simulink library "commeqprivlib"  (Simulink 6.0)
settings: Solver=ode45  SolverMode=SingleTasking  StartTime=0.0  StopTime=10.0  RelTol=1e-3
undefined symbols (not defined in the file or in its folder): bias, delay, incMu, lambda, leakage, maxMu, minMu, nFwdTaps, nSamp, nTaps, Rows, sigConst, stepSize
libraries: commeqprivlib x11, dspsigattribs x9, dspsigops x8, simulink x7, dspmtrx3 x5, dspindex x2, dspsrcs4 x2, dspbuff3 x1, dspstat3 x1
settings Model: Creator=skeene  LastModifiedBy=mclark  ProdHWDeviceType=Specified
settings DataIOCC: SignalLoggingName=logsOut
settings OptimizationCC: BooleanDataType=off
settings DebuggingCC: CheckExecutionContextPreStartOutputMsg=on  CheckExecutionContextRuntimeOutputMsg=on  SolverPrmCheckMsg=none
settings HardwareCC: ProdHWDeviceType=Specified  TargetUnknown=on
settings ModelReferenceCC: UpdateModelReferenceTargets=IfOutOfDate
settings GRTTargetCC: LifeSpan=inf
settings SFSimCC: SFSimApplyToAllLibs=on  SFSimBuildMode=Incremental

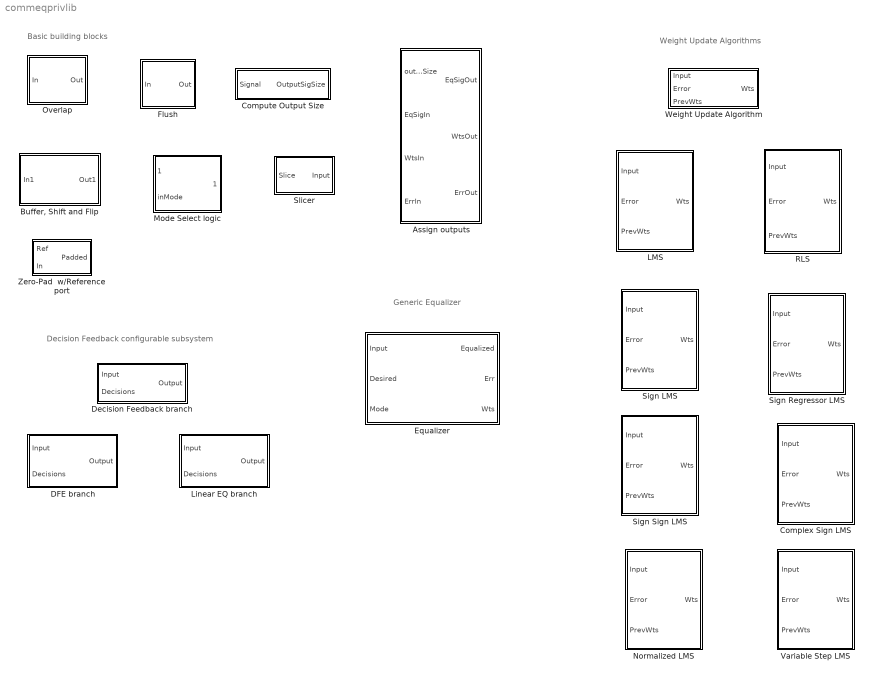
== system commeqprivlib ==
  note: Basic building blocks
  note: Decision Feedback configurable subsystem
  note: Generic Equalizer
  note: Weight Update Algorithms
  Assign outputs : Subsystem  EnableExecutionContextPropagation=on
  "Buffer, Shift and Flip" : Subsystem  EnableExecutionContextPropagation=on
  Complex Sign LMS : Subsystem  EnableExecutionContextPropagation=on
  Compute Output Size : Subsystem  EnableExecutionContextPropagation=on
  DFE branch : Subsystem  EnableExecutionContextPropagation=on
  Decision Feedback branch : Subsystem  BlockChoice=DFE branch  EnableExecutionContextPropagation=on
      settings: TemplateBlock=self  MemberBlocks=DFE branch,Linear EQ branch
  "Equalizer " : Subsystem  EnableExecutionContextPropagation=on  mask{eqType=Linear, alg=LMS}
      mask prompts: eqType "Equalizer type"; alg "Weight update algorithm"
      mask init:
      | commblkeq
      mask StyleString: popup(Linear|DFE),popup(LMS|RLS|Sign LMS|Sign Regressor LMS|Sign Sign LMS|Complex Sign LMS|Normalized LMS|Variable Step LMS)
      mask CallbackString: commblkeq|commblkeq
  Flush : Subsystem  EnableExecutionContextPropagation=on
  LMS : Subsystem  EnableExecutionContextPropagation=on
  Linear EQ branch : Subsystem  EnableExecutionContextPropagation=on
  Mode Select logic : Subsystem  EnableExecutionContextPropagation=on
  Normalized LMS : Subsystem  EnableExecutionContextPropagation=on
  Overlap : Subsystem  EnableExecutionContextPropagation=on
  RLS : Subsystem  EnableExecutionContextPropagation=on
  Sign LMS : Subsystem  EnableExecutionContextPropagation=on
  Sign Regressor LMS : Subsystem  EnableExecutionContextPropagation=on
  Sign Sign LMS : Subsystem  EnableExecutionContextPropagation=on
  Slicer : Subsystem  Orientation=left  EnableExecutionContextPropagation=on
  Variable Step LMS : Subsystem  EnableExecutionContextPropagation=on
  Weight Update Algorithm : Subsystem  BlockChoice=LMS  EnableExecutionContextPropagation=on
      settings: TemplateBlock=self  MemberBlocks=Complex Sign LMS,LMS,Normalized LMS,RLS,Sign LMS,Sign Regressor LMS,Sign Sign LMS,Variable Step LMS
  Zero-Pad  w/Reference port : Subsystem  EnableExecutionContextPropagation=on

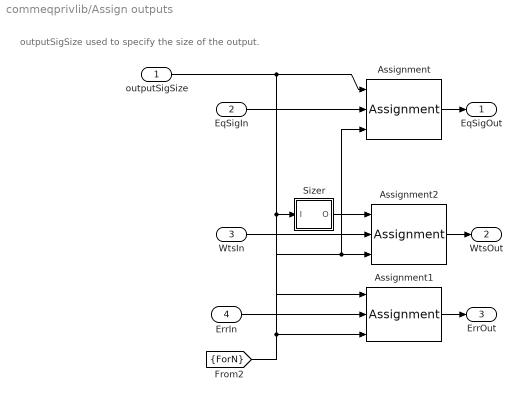
== system commeqprivlib/Assign outputs ==
  note: outputSigSize used to specify
      | the size of the output.
  outputSigSize : Inport  LatchInput=off
  EqSigIn : Inport  Port=2  LatchInput=off
  WtsIn : Inport  Port=3  LatchInput=off
  ErrIn : Inport  Port=4  LatchInput=off
  Assignment : Assignment  IndexMode=Zero-based  ElementSrc=External  Rows=-1  ColumnSrc=External  DiagnosticForDimensions=Error
  Assignment1 : Assignment  IndexMode=Zero-based  ElementSrc=External  Rows=-1  ColumnSrc=External  DiagnosticForDimensions=Error
  Assignment2 : Assignment  InputType=Matrix  IndexMode=Zero-based  ElementSrc=External  Rows=-1  ColumnSrc=External  DiagnosticForDimensions=Error
  Sizer : Subsystem  EnableExecutionContextPropagation=on
  EqSigOut : Outport
  WtsOut : Outport  Port=2
  ErrOut : Outport  Port=3
  wires:
  outputSigSize/1 -> Sizer/1(I), Assignment1/1, Assignment/1
  [ForN] -> Assignment1/3, Assignment/3, Assignment2/3
  Sizer/1(O) -> Assignment2/1
  EqSigIn/1 -> Assignment/2
  WtsIn/1 -> Assignment2/2
  ErrIn/1 -> Assignment1/2
  Assignment/1 -> EqSigOut/1
  Assignment2/1 -> WtsOut/1
  Assignment1/1 -> ErrOut/1

== system commeqprivlib/Buffer, Shift and Flip ==
  In1 : Inport  LatchInput=off
  Bias1 : Bias  Bias=0:nFwdTaps-1
  Flip : dspindex/Flip  dim=Columns
  Frame Status Conversion : dspsigattribs/Frame Status Conversion  growRefPort=off  outframe=Sample-based
  Gain : Gain  Gain=nSamp  SaturateOnIntegerOverflow=on
  Selector : Selector  IndexMode=Zero-based  ElementSrc=External  Elements=[1 3]
  Out1 : Outport
  wires:
  Frame Status Conversion/1 -> Out1/1
  In1/1 -> Selector/1
  Gain/1 -> Bias1/1
  [ForN] -> Gain/1
  Selector/1 -> Flip/1
  Flip/1 -> Frame Status Conversion/1
  Bias1/1 -> Selector/2

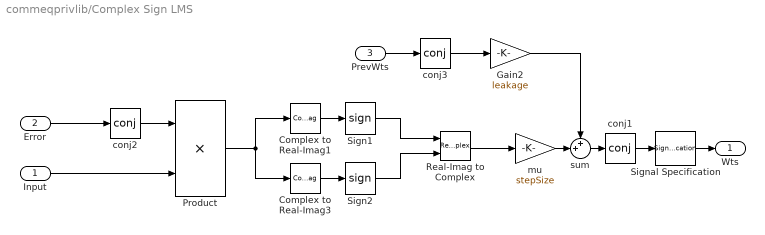
== system commeqprivlib/Complex Sign LMS ==
  Input : Inport  LatchInput=off
  Error : Inport  Port=2  LatchInput=off
  PrevWts : Inport  Port=3  LatchInput=off
  Complex to Real-Imag1 : ComplexToRealImag  Output=Real
  Complex to Real-Imag3 : ComplexToRealImag  Output=Imag
  Gain2 : Gain  Gain=leakage  SaturateOnIntegerOverflow=on
  Product : Product  SaturateOnIntegerOverflow=on
  Real-Imag to Complex : RealImagToComplex
  Sign1 : Signum
  Sign2 : Signum
  Signal Specification : SignalSpecification
      settings: SignalType=complex
  conj1 : Math  Operator=conj  SaturateOnIntegerOverflow=on
  conj2 : Math  Operator=conj  SaturateOnIntegerOverflow=on
  conj3 : Math  Operator=conj  SaturateOnIntegerOverflow=on
  mu : Gain  Gain=stepSize  SaturateOnIntegerOverflow=on
  sum : Sum  Inputs=++|  SaturateOnIntegerOverflow=on  InputSameDT=on
  Wts : Outport  InitialOutput=0
  wires:
  Product/1 -> Complex to Real-Imag1/1, Complex to Real-Imag3/1
  Complex to Real-Imag1/1 -> Sign1/1
  Gain2/1 -> sum/1
  PrevWts/1 -> conj3/1
  sum/1 -> conj1/1
  Input/1 -> Product/2
  Error/1 -> conj2/1
  mu/1 -> sum/2
  conj1/1 -> Signal Specification/1
  conj3/1 -> Gain2/1
  conj2/1 -> Product/1
  Signal Specification/1 -> Wts/1
  Real-Imag to Complex/1 -> mu/1
  Sign1/1 -> Real-Imag to Complex/1
  Complex to Real-Imag3/1 -> Sign2/1
  Sign2/1 -> Real-Imag to Complex/2

== system commeqprivlib/Compute Output Size ==
  Signal : Inport  LatchInput=off
  Downsample : dspsigops/Downsample  N=nSamp  phase=0  ic=0  smode=Force single rate  fmode=Maintain input frame rate
  Submatrix : dspmtrx3/Submatrix  RowSpan=Range of rows  RowStartMode=First  RowStartIndex=1  RowEndMode=Offset from last  RowEndIndex=nFwdTaps  ColSpan=Range of columns  ColStartMode=First  ColStartIndex=1  ColEndMode=Last  ColEndIndex=1
  OutputSigSize : Outport
  wires:
  Downsample/1 -> OutputSigSize/1
  Submatrix/1 -> Downsample/1
  Signal/1 -> Submatrix/1

== system commeqprivlib/DFE branch ==
  Input : Inport  LatchInput=off
  Decisions : Inport  Orientation=up  Port=2  LatchInput=off
  Delay Line : dspbuff3/Delay Line  Orientation=up  siz=nFdbkTaps  ic=0  directfeed=off
  Flip1 : dspindex/Flip  Orientation=up  dim=Columns
  Matrix Concatenation : simulink/Math Operations/Matrix Concatenation  numInports=2  catMethod=Vertical
  Output : Outport
  wires:
  Matrix Concatenation/1 -> Output/1
  Input/1 -> Matrix Concatenation/1
  Decisions/1 -> Delay Line/1
  Delay Line/1 -> Flip1/1
  Flip1/1 -> Matrix Concatenation/2

== system commeqprivlib/Decision Feedback branch ==
  Input : Inport  LatchInput=off
  Decisions : Inport  Port=2  LatchInput=off
  DFE branch : commeqprivlib/DFE branch  SimViewingDevice=off  DataTypeOverride=UseLocalSettings  MinMaxOverflowLogging=UseLocalSettings
      settings: Permissions=ReadWrite  RTWFcnNameOpts=Auto  RTWFileNameOpts=Auto
  Output : Outport
  wires:
  Input/1 -> DFE branch/1
  Decisions/1 -> DFE branch/2
  DFE branch/1 -> Output/1

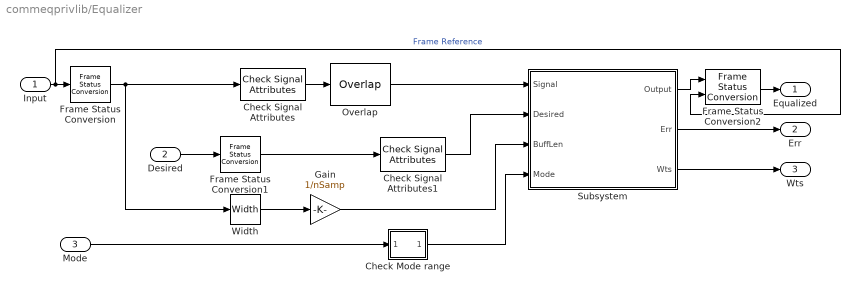
== system commeqprivlib/Equalizer  ==
  Input : Inport  LatchInput=off
  Desired : Inport  Port=2  LatchInput=off
  Mode : Inport  Port=3  LatchInput=off
  Check Mode range : Subsystem  EnableExecutionContextPropagation=on
  Check Signal Attributes : dspsigattribs/Check Signal Attributes  SigAttribCheckMethod=Does not match attributes exactly  Complexity=Complex  Frame=Ignore  DimsCheckMethod=Is not...  Dimensions=Full matrix (2-D)  DatatypeCheckMethod=Ignore  DatatypeGeneral=Boolean  DtypeFloatSpecific=Any floating-point  DtypeFixedSpecific=Any fixed-point  DtypeIntSpecific=Any integer  SampleMode=Ignore
  Check Signal Attributes1 : dspsigattribs/Check Signal Attributes  SigAttribCheckMethod=Does not match attributes exactly  Complexity=Complex  Frame=Ignore  DimsCheckMethod=Is not...  Dimensions=Full matrix (2-D)  DatatypeCheckMethod=Ignore  DatatypeGeneral=Boolean  DtypeFloatSpecific=Any floating-point  DtypeFixedSpecific=Any fixed-point  DtypeIntSpecific=Any integer  SampleMode=Ignore
  Frame Status Conversion : dspsigattribs/Frame Status Conversion  growRefPort=off  outframe=Frame-based
  Frame Status Conversion1 : dspsigattribs/Frame Status Conversion  growRefPort=off  outframe=Frame-based
  Frame Status Conversion2 : dspsigattribs/Frame Status Conversion  growRefPort=on  outframe=Frame-based
  Gain : Gain  Gain=1/nSamp  SaturateOnIntegerOverflow=on
  Overlap : commeqprivlib/Overlap
  Subsystem : Subsystem  EnableExecutionContextPropagation=on
  Width : Width  ShowAdditionalParam=on
  Equalized : Outport
  Err : Outport  Port=2
  Wts : Outport  Port=3
  wires:
  Frame Status Conversion/1 -> Width/1, Check Signal Attributes/1
  Frame Status Conversion1/1 -> Check Signal Attributes1/1
  Frame Status Conversion2/1 -> Equalized/1
  Subsystem/1(Output) -> Frame Status Conversion2/1
  Check Mode range/1("  ") -> Subsystem/4(Mode)
  Subsystem/3(Wts) -> Wts/1
  Subsystem/2(Err) -> Err/1
  Mode/1 -> Check Mode range/1("        ")
  Gain/1 -> Subsystem/3(BuffLen)
  Overlap/1 -> Subsystem/1(Signal)
  Desired/1 -> Frame Status Conversion1/1
  Input/1 -> Frame Status Conversion/1, Frame Status Conversion2/2  "Frame Reference"
  Width/1 -> Gain/1
  Check Signal Attributes1/1 -> Subsystem/2(Desired)
  Check Signal Attributes/1 -> Overlap/1

== system commeqprivlib/Flush ==
  note: This subsytem appends delay
      | samples to the reference signal.
      | The purpose of this is to flush out the
      | final samples from the delay block
      | that follows this subsystem.
  In : Inport  LatchInput=off
  Delay2 : dspsigops/Delay  Orientation=left  dly_unit=Samples  delay=delay  ic_detail=off  dif_ic_for_ch=off  dif_ic_for_dly=off  ic=0  reset_popup=None
  Matrix Concatenation : simulink/Math Operations/Matrix Concatenation  numInports=2  catMethod=Vertical
  Signal Specification : simulink/Signal Attributes/Signal Specification  Orientation=up  D=[delay 1]  Ts=-1  DataType=auto  OutDataType=sfix(16)  OutScaling=2^0
      settings: SignalType=auto  SamplingMode=auto
  Submatrix : dspmtrx3/Submatrix  Orientation=down  RowSpan=Range of rows  RowStartMode=Offset from last  RowStartIndex=delay-1  RowEndMode=Last  RowEndIndex=1  ColSpan=Range of columns  ColStartMode=First  ColStartIndex=1  ColEndMode=Last  ColEndIndex=1
  Out : Outport
  wires:
  Submatrix/1 -> Delay2/1
  Delay2/1 -> Signal Specification/1
  Matrix Concatenation/1 -> Out/1, Submatrix/1
  In/1 -> Matrix Concatenation/1
  Signal Specification/1 -> Matrix Concatenation/2

== system commeqprivlib/LMS ==
  Input : Inport  LatchInput=off
  Error : Inport  Port=2  LatchInput=off
  PrevWts : Inport  Port=3  LatchInput=off
  Gain2 : Gain  Gain=leakage  SaturateOnIntegerOverflow=on
  Product : Product  SaturateOnIntegerOverflow=on
  conj : Math  Operator=conj  SaturateOnIntegerOverflow=on
  mu : Gain  Gain=stepSize  SaturateOnIntegerOverflow=on
  sum : Sum  Inputs=++|  SaturateOnIntegerOverflow=on  InputSameDT=on
  Wts : Outport  InitialOutput=0
  wires:
  mu/1 -> Product/1
  Error/1 -> mu/1
  conj/1 -> Product/2
  Input/1 -> conj/1
  sum/1 -> Wts/1
  Product/1 -> sum/2
  PrevWts/1 -> Gain2/1
  Gain2/1 -> sum/1

== system commeqprivlib/Linear EQ branch ==
  note: There is no feedback in a linear equalizer
  Input : Inport  LatchInput=off
  Decisions : Inport  Orientation=up  Port=2  LatchInput=off
  Terminator : Terminator
      settings: Orientation=up
  Output : Outport
  wires:
  Decisions/1 -> Terminator/1
  Input/1 -> Output/1

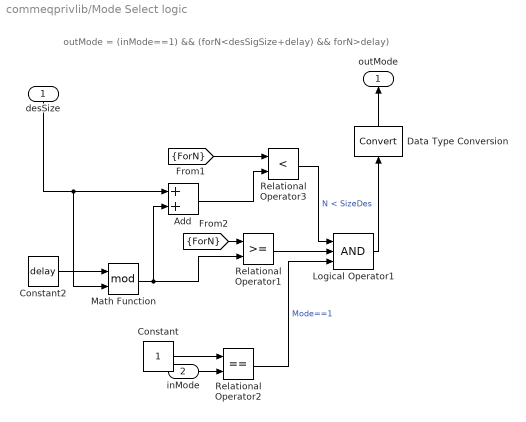
== system commeqprivlib/Mode Select logic ==
  note: outMode = (inMode==1) && (forN<desSigSize+delay) && forN>delay)
  desSize : Inport  Orientation=down  LatchInput=off
  inMode : Inport  Port=2  LatchInput=off
  Add : Sum  OutScaling=2^-10
  Constant : Constant
  Constant2 : Constant  Value=delay
  Data Type Conversion : DataTypeConversion  Orientation=up  OutDataTypeMode=double
  Logical Operator1 : Logic  Inputs=3  AllPortsSameDT=off  OutDataTypeMode=Boolean
  Math Function : Math  Operator=mod  SaturateOnIntegerOverflow=on
  Relational Operator1 : RelationalOperator  LogicOutDataTypeMode=Boolean
  Relational Operator2 : RelationalOperator  Operator===  LogicOutDataTypeMode=Boolean
  Relational Operator3 : RelationalOperator  Operator=<  LogicOutDataTypeMode=Boolean
  outMode : Outport  Orientation=up
  wires:
  inMode/1 -> Relational Operator2/2
  desSize/1 -> Add/1, Math Function/2
  Data Type Conversion/1 -> outMode/1
  Logical Operator1/1 -> Data Type Conversion/1
  Relational Operator3/1 -> Logical Operator1/1  "N < SizeDes"
  [ForN] -> Relational Operator3/1
  Constant/1 -> Relational Operator2/1
  Relational Operator2/1 -> Logical Operator1/3  "Mode==1"
  [ForN] -> Relational Operator1/1
  Relational Operator1/1 -> Logical Operator1/2
  Add/1 -> Relational Operator3/2
  Math Function/1 -> Add/2, Relational Operator1/2
  Constant2/1 -> Math Function/1

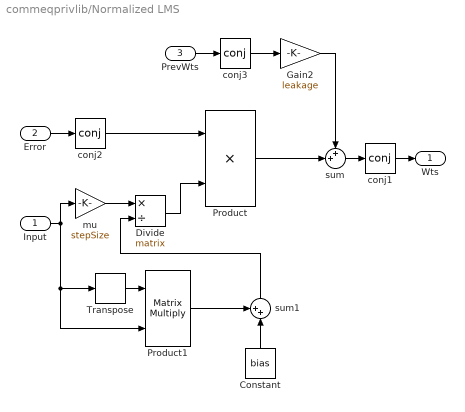
== system commeqprivlib/Normalized LMS ==
  Input : Inport  LatchInput=off
  Error : Inport  Port=2  LatchInput=off
  PrevWts : Inport  Port=3  LatchInput=off
  Constant : Constant  Orientation=up  Value=bias
  Divide : Product  Inputs=*/  Multiplication=Matrix(*)  OutScaling=2^-10
  Gain2 : Gain  Gain=leakage  SaturateOnIntegerOverflow=on
  Product : Product  SaturateOnIntegerOverflow=on
  Product1 : Product  Multiplication=Matrix(*)  SaturateOnIntegerOverflow=on
  Transpose : dspmtrx3/Transpose  Hermitian=on
  conj1 : Math  Operator=conj  SaturateOnIntegerOverflow=on
  conj2 : Math  Operator=conj  SaturateOnIntegerOverflow=on
  conj3 : Math  Operator=conj  SaturateOnIntegerOverflow=on
  mu : Gain  Gain=stepSize  SaturateOnIntegerOverflow=on
  sum : Sum  Inputs=++|  SaturateOnIntegerOverflow=on  InputSameDT=on
  sum1 : Sum  Orientation=up  Inputs=++|  SaturateOnIntegerOverflow=on  InputSameDT=on
  Wts : Outport  InitialOutput=0
  wires:
  conj1/1 -> Wts/1
  conj3/1 -> Gain2/1
  Error/1 -> conj2/1
  sum/1 -> conj1/1
  Product/1 -> sum/2
  PrevWts/1 -> conj3/1
  Gain2/1 -> sum/1
  conj2/1 -> Product/1
  Transpose/1 -> Product1/1
  Input/1 -> Product1/2, Transpose/1, mu/1
  Constant/1 -> sum1/2
  Product1/1 -> sum1/1
  sum1/1 -> Divide/2
  Divide/1 -> Product/2
  mu/1 -> Divide/1

== system commeqprivlib/Overlap ==
  note: This subsystem appends nTaps samples
      | to the input signal. The purpose of this is to remember
      | the previous nTaps sampes, as they are needed to
      | compute the current weights.
  In : Inport  LatchInput=off
  Delay2 : dspsigops/Delay  Orientation=left  dly_unit=Samples  delay=nFwdTaps  ic_detail=off  dif_ic_for_ch=off  dif_ic_for_dly=off  ic=0  reset_popup=None
  Matrix Concatenation : simulink/Math Operations/Matrix Concatenation  numInports=2  catMethod=Vertical
  Signal Specification : simulink/Signal Attributes/Signal Specification  Orientation=down  D=[nFwdTaps 1]  Ts=-1  DataType=auto  OutDataType=sfix(16)  OutScaling=2^0
      settings: SignalType=auto  SamplingMode=auto
  Submatrix : dspmtrx3/Submatrix  Orientation=up  RowSpan=Range of rows  RowStartMode=Offset from last  RowStartIndex=nFwdTaps-1  RowEndMode=Last  RowEndIndex=1  ColSpan=Range of columns  ColStartMode=First  ColStartIndex=1  ColEndMode=Last  ColEndIndex=1
  Out : Outport
  wires:
  In/1 -> Matrix Concatenation/2
  Submatrix/1 -> Delay2/1
  Delay2/1 -> Signal Specification/1
  Matrix Concatenation/1 -> Out/1, Submatrix/1
  Signal Specification/1 -> Matrix Concatenation/1

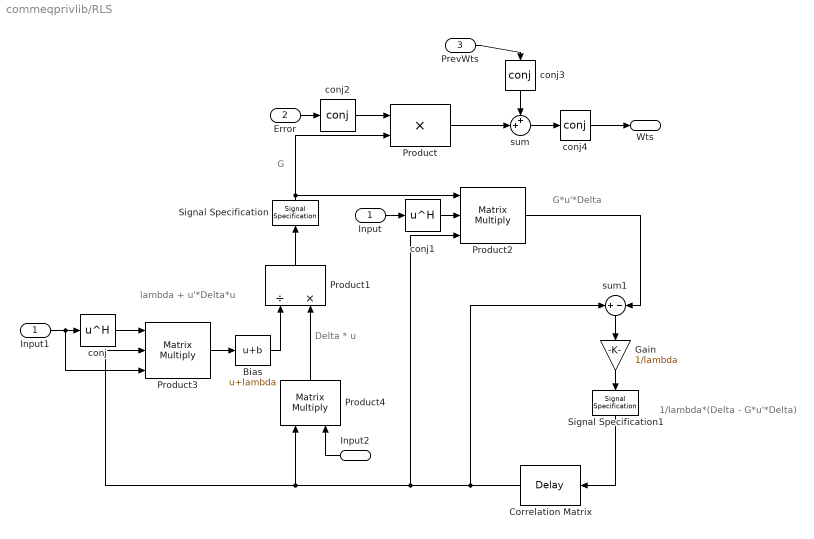
== system commeqprivlib/RLS ==
  note: G
  note: lambda + u'*Delta*u
  note: G*u'*Delta
  note: 1/lambda*(Delta - G*u'*Delta)
  note: Delta * u
  Input : Inport  LatchInput=off
  Error : Inport  Port=2  LatchInput=off
  PrevWts : Inport  Port=3  LatchInput=off
  Bias : Bias  Bias=lambda
  Correlation Matrix : dspsigops/Delay  Orientation=left  dly_unit=Samples  delay=1  ic_detail=on  dif_ic_for_ch=on  dif_ic_for_dly=off  ic=invCorr  reset_popup=None
  Gain : Gain  Orientation=down  Gain=1/lambda
  Input1 : InportShadow  LatchInput=off
  Input2 : InportShadow  Orientation=left  LatchInput=off
  Product : Product  SaturateOnIntegerOverflow=on
  Product1 : Product  Orientation=up  Inputs=/*  SaturateOnIntegerOverflow=on
  Product2 : Product  Inputs=3  Multiplication=Matrix(*)  SaturateOnIntegerOverflow=on
  Product3 : Product  Inputs=3  Multiplication=Matrix(*)  SaturateOnIntegerOverflow=on
  Product4 : Product  Orientation=up  Multiplication=Matrix(*)  SaturateOnIntegerOverflow=on
  Signal Specification : SignalSpecification  Orientation=up  Dimensions=[nTaps 1]
  Signal Specification1 : SignalSpecification  Orientation=down  Dimensions=[nTaps nTaps]
  conj : Math  Operator=hermitian  SaturateOnIntegerOverflow=on
  conj1 : Math  Operator=hermitian  SaturateOnIntegerOverflow=on
  conj2 : Math  Operator=conj  SaturateOnIntegerOverflow=on
  conj3 : Math  Orientation=down  Operator=conj  SaturateOnIntegerOverflow=on
  conj4 : Math  Operator=conj  SaturateOnIntegerOverflow=on
  sum : Sum  Inputs=++|  SaturateOnIntegerOverflow=on  InputSameDT=on
  sum1 : Sum  Orientation=down  Inputs=+-  SaturateOnIntegerOverflow=on  InputSameDT=on
  Wts : Outport  InitialOutput=0
  wires:
  Error/1 -> conj2/1
  Product1/1 -> Signal Specification/1
  Product/1 -> sum/2
  PrevWts/1 -> conj3/1
  sum/1 -> conj4/1
  Input/1 -> conj1/1
  conj/1 -> Product3/1
  Input1/1 -> conj/1, Product3/3
  Product3/1 -> Bias/1
  Bias/1 -> Product1/1
  Product4/1 -> Product1/2
  Input2/1 -> Product4/2
  Correlation Matrix/1 -> Product4/1, Product3/2, Product2/3, sum1/1
  Product2/1 -> sum1/2
  sum1/1 -> Gain/1
  Gain/1 -> Signal Specification1/1
  conj1/1 -> Product2/2
  conj2/1 -> Product/1
  Signal Specification/1 -> Product/2, Product2/1
  Signal Specification1/1 -> Correlation Matrix/1
  conj3/1 -> sum/1
  conj4/1 -> Wts/1

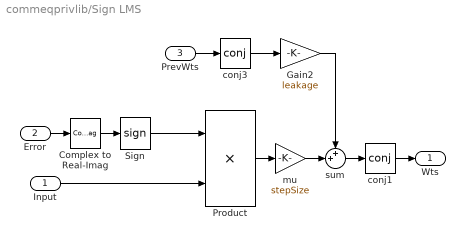
== system commeqprivlib/Sign LMS ==
  Input : Inport  LatchInput=off
  Error : Inport  Port=2  LatchInput=off
  PrevWts : Inport  Port=3  LatchInput=off
  Complex to Real-Imag : ComplexToRealImag  Output=Real
  Gain2 : Gain  Gain=leakage  SaturateOnIntegerOverflow=on
  Product : Product  SaturateOnIntegerOverflow=on
  Sign : Signum
  conj1 : Math  Operator=conj  SaturateOnIntegerOverflow=on
  conj3 : Math  Operator=conj  SaturateOnIntegerOverflow=on
  mu : Gain  Gain=stepSize  SaturateOnIntegerOverflow=on
  sum : Sum  Inputs=++|  SaturateOnIntegerOverflow=on  InputSameDT=on
  Wts : Outport  InitialOutput=0
  wires:
  Gain2/1 -> sum/1
  PrevWts/1 -> conj3/1
  Product/1 -> mu/1
  sum/1 -> conj1/1
  Input/1 -> Product/2
  Error/1 -> Complex to Real-Imag/1
  Complex to Real-Imag/1 -> Sign/1
  Sign/1 -> Product/1
  conj3/1 -> Gain2/1
  conj1/1 -> Wts/1
  mu/1 -> sum/2

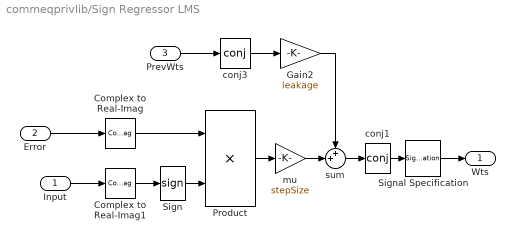
== system commeqprivlib/Sign Regressor LMS ==
  Input : Inport  LatchInput=off
  Error : Inport  Port=2  LatchInput=off
  PrevWts : Inport  Port=3  LatchInput=off
  Complex to Real-Imag : ComplexToRealImag  Output=Real
  Complex to Real-Imag1 : ComplexToRealImag  Output=Real
  Gain2 : Gain  Gain=leakage  SaturateOnIntegerOverflow=on
  Product : Product  SaturateOnIntegerOverflow=on
  Sign : Signum
  Signal Specification : SignalSpecification
      settings: SignalType=complex
  conj1 : Math  Operator=conj  SaturateOnIntegerOverflow=on
  conj3 : Math  Operator=conj  SaturateOnIntegerOverflow=on
  mu : Gain  Gain=stepSize  SaturateOnIntegerOverflow=on
  sum : Sum  Inputs=++|  SaturateOnIntegerOverflow=on  InputSameDT=on
  Wts : Outport  InitialOutput=0
  wires:
  Error/1 -> Complex to Real-Imag/1
  Input/1 -> Complex to Real-Imag1/1
  sum/1 -> conj1/1
  Product/1 -> mu/1
  PrevWts/1 -> conj3/1
  Gain2/1 -> sum/1
  Complex to Real-Imag/1 -> Product/1
  Complex to Real-Imag1/1 -> Sign/1
  Sign/1 -> Product/2
  conj3/1 -> Gain2/1
  conj1/1 -> Signal Specification/1
  mu/1 -> sum/2
  Signal Specification/1 -> Wts/1

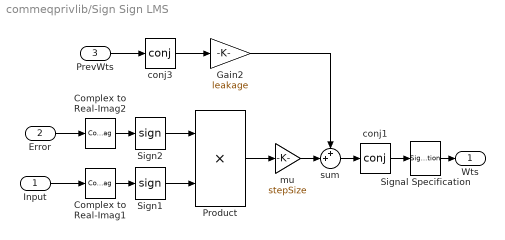
== system commeqprivlib/Sign Sign LMS ==
  Input : Inport  LatchInput=off
  Error : Inport  Port=2  LatchInput=off
  PrevWts : Inport  Port=3  LatchInput=off
  Complex to Real-Imag1 : ComplexToRealImag  Output=Real
  Complex to Real-Imag2 : ComplexToRealImag  Output=Real
  Gain2 : Gain  Gain=leakage  SaturateOnIntegerOverflow=on
  Product : Product  SaturateOnIntegerOverflow=on
  Sign1 : Signum
  Sign2 : Signum
  Signal Specification : SignalSpecification
      settings: SignalType=complex
  conj1 : Math  Operator=conj  SaturateOnIntegerOverflow=on
  conj3 : Math  Operator=conj  SaturateOnIntegerOverflow=on
  mu : Gain  Gain=stepSize  SaturateOnIntegerOverflow=on
  sum : Sum  Inputs=++|  SaturateOnIntegerOverflow=on  InputSameDT=on
  Wts : Outport  InitialOutput=0
  wires:
  sum/1 -> conj1/1
  PrevWts/1 -> conj3/1
  Gain2/1 -> sum/1
  conj3/1 -> Gain2/1
  conj1/1 -> Signal Specification/1
  mu/1 -> sum/2
  Product/1 -> mu/1
  Error/1 -> Complex to Real-Imag2/1
  Complex to Real-Imag2/1 -> Sign2/1
  Sign2/1 -> Product/1
  Input/1 -> Complex to Real-Imag1/1
  Complex to Real-Imag1/1 -> Sign1/1
  Sign1/1 -> Product/2
  Signal Specification/1 -> Wts/1

== system commeqprivlib/Slicer ==
  Input : Inport  Orientation=left  LatchInput=off
  Linear Demodulator : Subsystem  Orientation=left  EnableExecutionContextPropagation=on
  Linear Modulator : Lookup  Orientation=left  DialogController=Simulink.DDGSource  InputValues=[1:length(sigConst)]  OutputValues=sigConst  LookUpMeth=Use Input Nearest  SaturateOnIntegerOverflow=on
  Slice : Outport  Orientation=left
  wires:
  Linear Modulator/1 -> Slice/1
  Input/1 -> Linear Demodulator/1(In1)
  Linear Demodulator/1(Out1) -> Linear Modulator/1

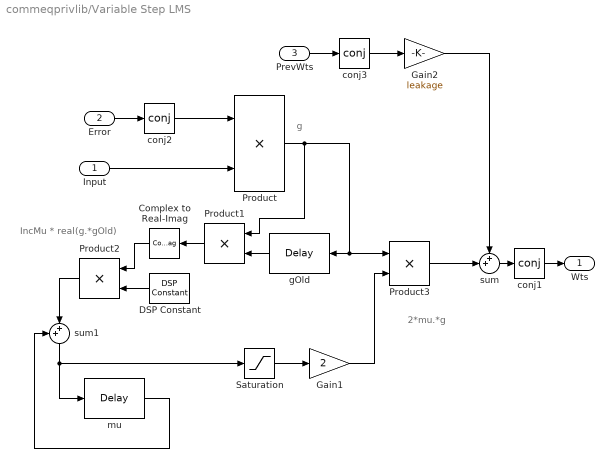
== system commeqprivlib/Variable Step LMS ==
  note: g
  note: IncMu * real(g.*gOld)
  note: 2*mu.*g
  Input : Inport  LatchInput=off
  Error : Inport  Port=2  LatchInput=off
  PrevWts : Inport  Port=3  LatchInput=off
  Complex to Real-Imag : ComplexToRealImag  Orientation=left  Output=Real
  DSP Constant : dspsrcs4/DSP Constant  Orientation=left  Value=incMu  SampleMode=Discrete  discreteOutput=Sample-based  continuousOutput=Sample-based  sampTime=-1  framePeriod=2  dataType=Inherit from 'Constant value'  wordLen=16  udDataType=sfix(16)  fracBitsMode=Best precision  numFracBits=15  InterpretAs1D=-inf  Ts=-inf  FramebasedOutput=-inf
  Gain1 : Gain  Gain=2  SaturateOnIntegerOverflow=on
  Gain2 : Gain  Gain=leakage  SaturateOnIntegerOverflow=on
  Product : Product  SaturateOnIntegerOverflow=on
  Product1 : Product  Orientation=left  SaturateOnIntegerOverflow=on
  Product2 : Product  Orientation=left  SaturateOnIntegerOverflow=on
  Product3 : Product  SaturateOnIntegerOverflow=on
  Saturation : Saturate  UpperLimit=maxMu  LowerLimit=minMu
  conj1 : Math  Operator=conj  SaturateOnIntegerOverflow=on
  conj2 : Math  Operator=conj  SaturateOnIntegerOverflow=on
  conj3 : Math  Operator=conj  SaturateOnIntegerOverflow=on
  gOld : dspsigops/Delay  Orientation=left  dly_unit=Samples  delay=1  ic_detail=on  dif_ic_for_ch=off  dif_ic_for_dly=off  ic=0  reset_popup=None
  mu : dspsigops/Delay  dly_unit=Samples  delay=1  ic_detail=on  dif_ic_for_ch=off  dif_ic_for_dly=off  ic=initMu  reset_popup=None
  sum : Sum  Inputs=++|  SaturateOnIntegerOverflow=on  InputSameDT=on
  sum1 : Sum  Orientation=down  Inputs=++|  SaturateOnIntegerOverflow=on  InputSameDT=on
  Wts : Outport  InitialOutput=0
  wires:
  Gain2/1 -> sum/1
  PrevWts/1 -> conj3/1
  Product/1 -> Product1/1, Product3/1, gOld/1
  sum/1 -> conj1/1
  conj3/1 -> Gain2/1
  conj1/1 -> Wts/1
  Input/1 -> Product/2
  Error/1 -> conj2/1
  conj2/1 -> Product/1
  DSP Constant/1 -> Product2/2
  gOld/1 -> Product1/2
  Product1/1 -> Complex to Real-Imag/1
  Complex to Real-Imag/1 -> Product2/1
  sum1/1 -> mu/1, Saturation/1
  mu/1 -> sum1/1
  Product2/1 -> sum1/2
  Gain1/1 -> Product3/2
  Product3/1 -> sum/2
  Saturation/1 -> Gain1/1

== system commeqprivlib/Weight Update Algorithm ==
  Input : Inport  LatchInput=off
  Error : Inport  Port=2  LatchInput=off
  PrevWts : Inport  Port=3  LatchInput=off
  LMS : commeqprivlib/LMS
  Wts : Outport
  wires:
  Input/1 -> LMS/1
  Error/1 -> LMS/2
  PrevWts/1 -> LMS/3
  LMS/1 -> Wts/1

== system commeqprivlib/Zero-Pad  w/Reference port ==
  Ref : Inport  LatchInput=off
  In : Inport  Port=2  LatchInput=off
  Assignment : Assignment  IndexMode=Zero-based  ElementSrc=External  Rows=-1  ColumnSrc=External  DiagnosticForDimensions=Error
  Constant Ramp : dspsrcs4/Constant Ramp  L=Rows  Slope=1  dataType=Same as input  wordLen=16  udDataType=sfix(16)  fracBitsMode=Best precision  numFracBits=15  Offset=0
  Gain : Gain  Gain=0
  Padded : Outport
  wires:
  Ref/1 -> Gain/1
  In/1 -> Assignment/2, Constant Ramp/1
  Gain/1 -> Assignment/1
  Assignment/1 -> Padded/1
  Constant Ramp/1 -> Assignment/3

== system commeqprivlib/Assign outputs/Sizer ==
  I : Inport  LatchInput=off
  Constant : Constant  Value=ones(1,nTaps)  VectorParams1D=off
  Product : Product  Multiplication=Matrix(*)  SaturateOnIntegerOverflow=on  RndMeth=Zero
  Transpose : dspmtrx3/Transpose  Hermitian=off
  O : Outport
  wires:
  Transpose/1 -> O/1
  I/1 -> Product/1
  Product/1 -> Transpose/1
  Constant/1 -> Product/2

== system commeqprivlib/Equalizer /Check Mode range ==
  "        " : Inport  LatchInput=off
  Check  Static Range : simulink/Model Verification/Check  Static Range  Description=0 <= u <= 1  max=1  max_included=on  min=0  min_included=on  enabled=on  callback=error('Mode input must be 0 or 1.')  stopWhenAssertionFail=on  export=off  icon=graphic
  Check Input  Resolution : simulink/Model Verification/Check Input  Resolution  Description=-Inf < u < +Inf  resolution=1  enabled=on  callback=error('Mode input must be 0 or 1.')  stopWhenAssertionFail=on  export=off
  Check Signal Attributes1 : dspsigattribs/Check Signal Attributes  SigAttribCheckMethod=Does not match attributes exactly  Complexity=Real  Frame=Ignore  DimsCheckMethod=Is...  Dimensions=Scalar (1-D or 2-D)  DatatypeCheckMethod=Ignore  DatatypeGeneral=Boolean  DtypeFloatSpecific=Any floating-point  DtypeFixedSpecific=Any fixed-point  DtypeIntSpecific=Any integer  SampleMode=Ignore
  "  " : Outport
  wires:
  "        "/1 -> Check  Static Range/1, Check Input  Resolution/1, Check Signal Attributes1/1
  Check Signal Attributes1/1 -> "  "/1

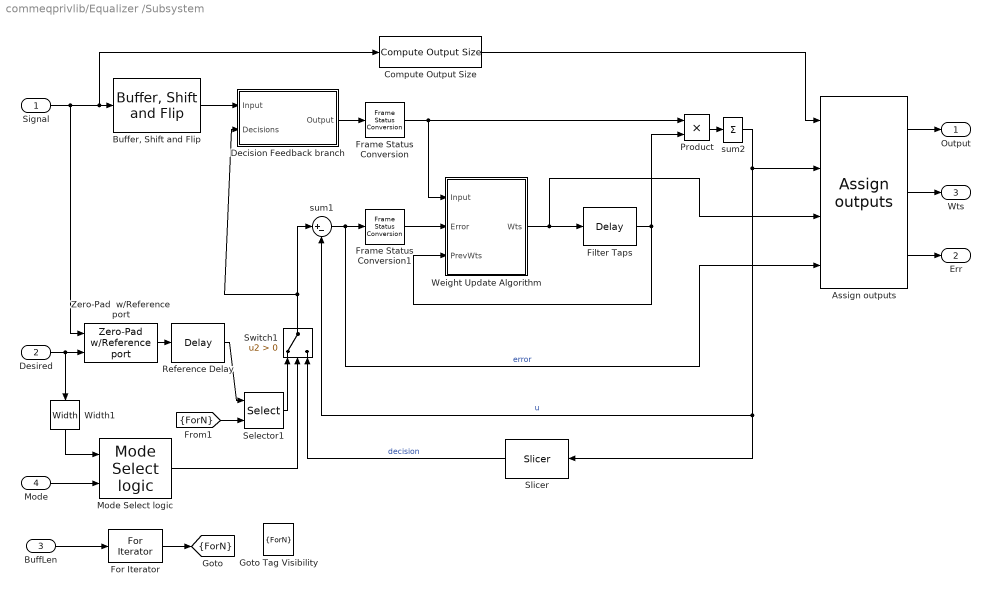
== system commeqprivlib/Equalizer /Subsystem ==
  Signal : Inport  LatchInput=off
  Desired : Inport  Port=2  LatchInput=off
  BuffLen : Inport  Port=3  LatchInput=off
  Mode : Inport  Port=4  LatchInput=off
  Assign outputs : commeqprivlib/Assign outputs
  "Buffer, Shift and Flip" : commeqprivlib/Buffer, Shift and Flip
  Compute Output Size : commeqprivlib/Compute Output Size
  Decision Feedback branch : Subsystem  BlockChoice=Linear EQ branch  EnableExecutionContextPropagation=on
      settings: AttributesFormatString=%<BlockChoice>  TemplateBlock=commeqprivlib/Decision Feedback branch  MemberBlocks=DFE branch,Linear EQ branch
  Filter Taps : dspsigops/Delay  dly_unit=Samples  delay=1  ic_detail=on  dif_ic_for_ch=on  dif_ic_for_dly=off  ic=initWeights  reset_popup=None
  For Iterator : ForIterator  IterationSource=external  IterationLimit=4  IndexMode=Zero-based  IterationVariableDataType=double
  Frame Status Conversion : dspsigattribs/Frame Status Conversion  growRefPort=off  outframe=Sample-based
  Frame Status Conversion1 : dspsigattribs/Frame Status Conversion  growRefPort=off  outframe=Sample-based
  Goto Tag Visibility : GotoTagVisibility  GotoTag=ForN
  Mode Select logic : commeqprivlib/Mode Select logic
  Product : Product  SaturateOnIntegerOverflow=on
  Reference Delay : dspsigops/Delay  dly_unit=Samples  delay=delay  ic_detail=off  dif_ic_for_ch=off  dif_ic_for_dly=off  ic=0  reset_popup=None
  Selector1 : Selector  IndexMode=Zero-based  ElementSrc=External  Elements=[1 3]
  Slicer : commeqprivlib/Slicer  Orientation=left
  Switch1 : Switch  Orientation=up  Criteria=u2 > Threshold  SaturateOnIntegerOverflow=on
  Weight Update Algorithm : Subsystem  BlockChoice=LMS  EnableExecutionContextPropagation=on
      settings: AttributesFormatString=%<BlockChoice>  TemplateBlock=commeqprivlib/Weight Update Algorithm  MemberBlocks=Complex Sign LMS,LMS,Normalized LMS,RLS,Sign LMS,Sign Regressor LMS,Sign Sign LMS,Variable Step LMS
  Width1 : Width  Orientation=down  ShowAdditionalParam=on
  Zero-Pad  w/Reference port : commeqprivlib/Zero-Pad  w//Reference port
  sum1 : Sum  Inputs=|+-  SaturateOnIntegerOverflow=on  InputSameDT=on
  sum2 : Sum  Inputs=+  SaturateOnIntegerOverflow=on  InputSameDT=on
  Output : Outport
  Err : Outport  Port=2
  Wts : Outport  Port=3
  tag scope: ForN=scoped
  wires:
  [ForN] -> Selector1/2
  Width1/1 -> Mode Select logic/1
  Assign outputs/1 -> Output/1
  Compute Output Size/1 -> Assign outputs/1
  Mode Select logic/1 -> Switch1/2
  Mode/1 -> Mode Select logic/2
  Signal/1 -> Compute Output Size/1, "Buffer, Shift and Flip"/1, Zero-Pad  w/Reference port/1
  Slicer/1 -> Switch1/3  "decision"
  Assign outputs/2 -> Wts/1
  Switch1/1 -> Decision Feedback branch/2(Decisions), sum1/1
  Selector1/1 -> Switch1/1
  sum2/1 -> sum1/2, Slicer/1, Assign outputs/2  "u"
  Filter Taps/1 -> Product/2, Weight Update Algorithm/3(PrevWts)
  Weight Update Algorithm/1(Wts) -> Filter Taps/1, Assign outputs/3
  Product/1 -> sum2/1
  Assign outputs/3 -> Err/1
  For Iterator/1 -> [ForN]
  sum1/1 -> Frame Status Conversion1/1, Assign outputs/4  "error"
  BuffLen/1 -> For Iterator/1
  Decision Feedback branch/1(Output) -> Frame Status Conversion/1
  "Buffer, Shift and Flip"/1 -> Decision Feedback branch/1(Input)
  Frame Status Conversion/1 -> Product/1, Weight Update Algorithm/1(Input)
  Frame Status Conversion1/1 -> Weight Update Algorithm/2(Error)
  Reference Delay/1 -> Selector1/1
  Desired/1 -> Width1/1, Zero-Pad  w/Reference port/2
  Zero-Pad  w/Reference port/1 -> Reference Delay/1

== system commeqprivlib/Slicer/Linear Demodulator ==
  In1 : Inport  LatchInput=off
  Abs : Abs  SaturateOnIntegerOverflow=on
  Constellation : Constant  Value=sigConst  VectorParams1D=off
  Minimum : dspstat3/Minimum  fcn=Index  reset=None  roundingMode=Floor  overflowMode=off
  Sum : Sum  Inputs=|+-  SaturateOnIntegerOverflow=on
  Out1 : Outport
  wires:
  Minimum/1 -> Out1/1
  Constellation/1 -> Sum/2
  Sum/1 -> Abs/1
  Abs/1 -> Minimum/1
  In1/1 -> Sum/1

== system commeqprivlib/Equalizer /Subsystem/Decision Feedback branch ==
  Input : Inport  LatchInput=off
  Decisions : Inport  Port=2  LatchInput=off
  Linear EQ branch : commeqprivlib/Linear EQ branch
  Output : Outport
  wires:
  Input/1 -> Linear EQ branch/1
  Decisions/1 -> Linear EQ branch/2
  Linear EQ branch/1 -> Output/1

== system commeqprivlib/Equalizer /Subsystem/Weight Update Algorithm ==
  Input : Inport  LatchInput=off
  Error : Inport  Port=2  LatchInput=off
  PrevWts : Inport  Port=3  LatchInput=off
  LMS : commeqprivlib/LMS
  Wts : Outport
  wires:
  Input/1 -> LMS/1
  Error/1 -> LMS/2
  PrevWts/1 -> LMS/3
  LMS/1 -> Wts/1
